simulink model "eulerAnglePropagate"  (R2023b)
settings: Solver=VariableStepAuto  StartTime=0.0  StopTime=Tfinal  RelTol=1e-3
settings Model: Creator=stanforduser  LastModifiedBy=stanforduser

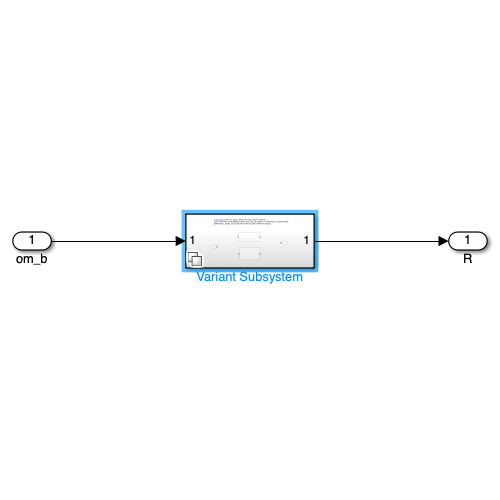
[thumbnail: Simulink's stored preview of the top-level diagram]
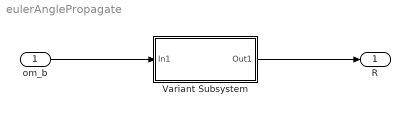
== system eulerAnglePropagate ==
  om_b : Inport
  Variant Subsystem : Subsystem  Variant=on
  R : Outport
  wires:
  om_b/1 -> Variant Subsystem/1(In1)
  Variant Subsystem/1(Out1) -> R/1

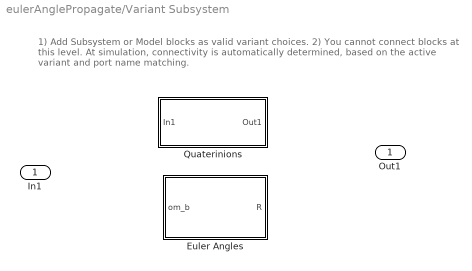
== system eulerAnglePropagate/Variant Subsystem ==
  note: 1) Add Subsystem or Model blocks as valid variant choices.
      | 2) You cannot connect blocks at this level. At simulation, connectivity is automatically
      | determined, based on the active variant and port name matching.
  In1 : Inport
  Euler Angles : Subsystem  VariantControl=Choice
  Quaterinions : Subsystem  VariantControl=true
  Out1 : Outport

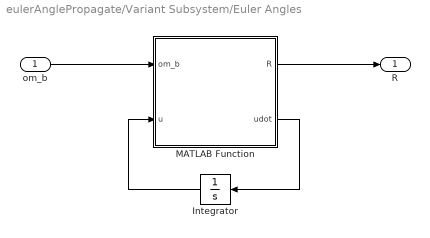
== system eulerAnglePropagate/Variant Subsystem/Euler Angles ==
  om_b : Inport
  Integrator : Integrator
  MATLAB Function : MATLAB Function  TreatAsAtomicUnit=on
  R : Outport
  wires:
  om_b/1 -> MATLAB Function/1(om_b)
  MATLAB Function/1(R) -> R/1
  Integrator/1 -> MATLAB Function/2(u)
  MATLAB Function/2(udot) -> Integrator/1

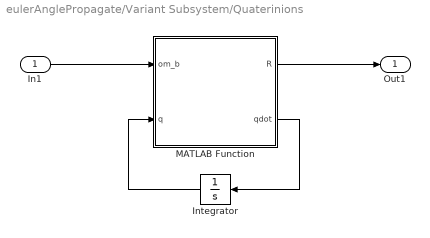
== system eulerAnglePropagate/Variant Subsystem/Quaterinions ==
  In1 : Inport
  Integrator : Integrator
  MATLAB Function : MATLAB Function  TreatAsAtomicUnit=on
  Out1 : Outport
  wires:
  In1/1 -> MATLAB Function/1(om_b)
  MATLAB Function/1(R) -> Out1/1
  Integrator/1 -> MATLAB Function/2(q)
  MATLAB Function/2(qdot) -> Integrator/1

== matlab function eulerAnglePropagate/Variant Subsystem/Euler Angles/MATLAB Function ==
  data: om_b input; u input; R output; udot output
function [R, udot] = eulerAnglePropagate(om_b, u)

% udot = zeros(size(u));

phi = u(1);
theta = u(2);
psi = u(3);

E_prime_inv = (1/sin(theta)) * [-sin(phi)*cos(theta), -cos(phi)*cos(theta), sin(theta);
                                cos(phi)*sin(theta), -sin(phi)*sin(theta), 0;
                                sin(phi), cos(phi), 0];

udot = E_prime_inv*om_b;


R = [cos(phi)*cos(psi) - sin(phi)*cos(theta)*sin(psi) , cos(phi)*sin(psi) + sin(phi)*cos(theta)*cos(psi), sin(phi)*sin(theta);
    -sin(phi)*cos(psi) - cos(phi)*cos(theta)*sin(psi), -sin(phi)*sin(psi) + cos(phi)*cos(theta)*cos(psi), cos(phi)*sin(theta);
    sin(theta)*sin(psi), -sin(theta)*cos(psi), cos(theta)];

== matlab function eulerAnglePropagate/Variant Subsystem/Quaterinions/MATLAB Function ==
  data: om_b input; q input; R output; qdot output
function [R, qdot] = eulerAnglePropagate(om_b, q)

% udot = zeros(size(u));

q0 = q(1);
q1 = q(2);
q2 = q(3);
q3 = q(4);
qvec = q(2:end);

W_prime = [-q1, q0, q3, -q2;
            -q2, -q3, q0, q1;
            -q3, q2, -q1, q0];

qdot = (1/2)*(W_prime.')*om_b;

% R = (q0^2 - norm(qvec)^2).*eye(3) + 2*qvec*qvec.T - 2*q0

R = [q0^2 + q1^2 - q2^2 - q3^2, 2*q1*q2 + 2*q0 + q3, 2*(q1*q3 - q0*q2);
    2*(q1*q2 - q0*q3), q0^2 - q1^2 + q2^2 - q3^2, 2*(q2*q3 + q0*q1);
    2*(q1*q3 + q0*q2), 2*(q2*q3 - q0*q1), q0^2 - q1^2 - q2^2 + q3^2];
